simulink model "CTR_Control_Simulation"  (R2018b)
settings: Solver=FixedStepAuto  StartTime=0.0  StopTime=20  FixedStep=0.05  RelTol=1e-3
libraries: simulink x1, dspinverses x1, powerlib_meascontrol x1
settings Model: Creator=mohsen  LastModifiedBy=Mohsen
settings SFSimCC: SimUseLocalCustomCode=off
settings RTWCC: RTWUseLocalCustomCode=off

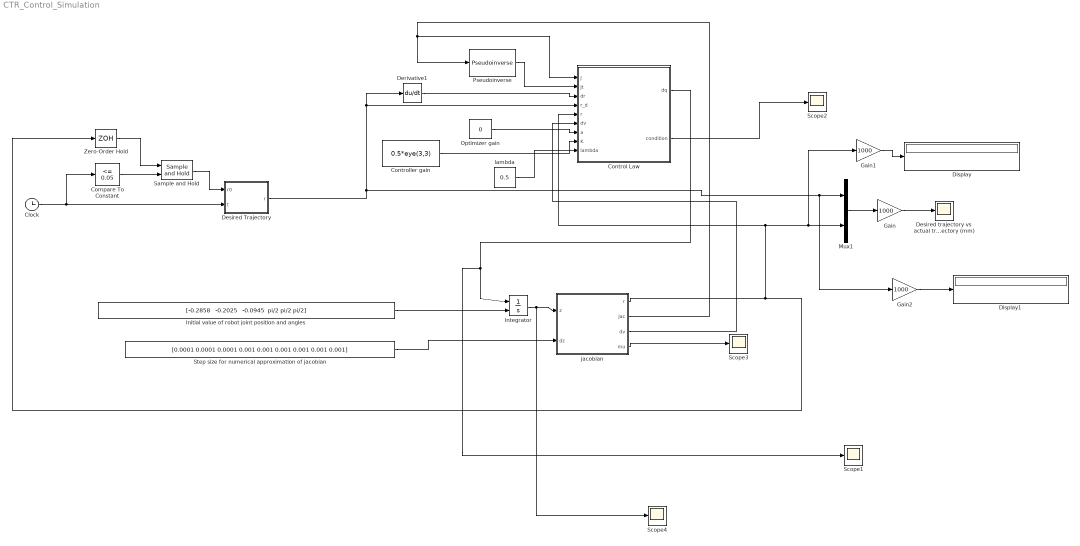
== system CTR_Control_Simulation ==
  Clock : Clock
  Compare To Constant : simulink/Logic and Bit Operations/Compare To Constant  relop=<=  const=0.05  OutDataTypeStr=boolean
  Control Law : MATLAB Function  TreatAsAtomicUnit=on
  Controller gain : Constant  Value=0.5*eye(3,3)
  Derivative1 : Derivative
  Desired Trajectory : MATLAB Function  TreatAsAtomicUnit=on
  Desired trajectory vs actual trajectory (mm) : Scope
  Display : Display
  Display1 : Display
  Gain : Gain  Gain=1000
  Gain1 : Gain  Gain=1000
  Gain2 : Gain  Gain=1000
  Initial value of robot joint position and angles : Constant  Value="[-0.2858   -0.2025   -0.0945  pi/2 pi/2 pi/2]"  VectorParams1D=off  SampleTime=-1
  Integrator : Integrator  InitialConditionSource=external  InitialCondition="[-0.2700   -0.1950   -0.0950    pi/2 pi/2 pi/2 ]"
  Mux1 : Mux  Inputs=2
  Optimizer gain : Constant  Value=0
  Pseudoinverse : dspinverses/Pseudoinverse  wanterr=off  SimulateUsing=Interpreted execution
      settings: SourceProductName=DSP System Toolbox  SourceProductBaseCode=DS
  Sample and Hold : powerlib_meascontrol/Additional Components/Sample and Hold  ic=0  Ts=0
      settings: SourceProductName=Simscape Electrical  SourceProductBaseCode=PS
  Scope{1..4} (4 alike) : Scope
  Step size for numerical approximation of jacobian : Constant  Value=[0.0001 0.0001 0.0001 0.001 0.001 0.001 0.001 0.001 0.001]
  Zero-Order Hold : ZeroOrderHold  SampleTime=5
  jacobian : MATLAB Function  TreatAsAtomicUnit=on
  lambda : Constant  Value=0.5
  wires:
  jacobian/2(Jac) -> Pseudoinverse/1, Control Law/1(J)
  Derivative1/1 -> Control Law/3(dr)
  Mux1/1 -> Gain/1
  Desired Trajectory/1(r) -> Control Law/4(r_d), Derivative1/1, Gain2/1, Mux1/1
  jacobian/1(r) -> Gain1/1, Mux1/2, Control Law/5(r), Zero-Order Hold/1
  Gain/1 -> Desired trajectory vs actual trajectory (mm)/1
  Pseudoinverse/1 -> Control Law/2(Jt)
  Control Law/1(dq) -> Scope1/1, Integrator/1
  Integrator/1 -> Scope4/1, jacobian/1(z)
  Step size for numerical approximation of jacobian/1 -> jacobian/2(dz)
  jacobian/3(dv) -> Control Law/6(dv)
  Optimizer gain/1 -> Control Law/7(a)
  jacobian/4(mu) -> Scope3/1
  Sample and Hold/1 -> Desired Trajectory/1(r0)
  Initial value of robot joint position and angles/1 -> Integrator/2
  Controller gain/1 -> Control Law/8(K)
  Clock/1 -> Compare To Constant/1, Desired Trajectory/2(t)
  Zero-Order Hold/1 -> Sample and Hold/1
  Compare To Constant/1 -> Sample and Hold/2
  Control Law/2(condition) -> Scope2/1
  lambda/1 -> Control Law/9(lambda)
  Gain1/1 -> Display/1
  Gain2/1 -> Display1/1

== matlab function CTR_Control_Simulation/Desired Trajectory ==
  data: r0 input; r output; t input
function r = fcn(r0, t)


if t>0.01
    %straight line -- set runtime to 5 sec and optimazer gain to 0.02 and
    %controller gain to 5*eye(3,3) and all inital angles to 0
    %Velocity=0.001;
    %r=r0+[-Velocity*t 2.*Velocity*t Velocity*t]';  
    
    %circle -- set runtime to 40 sec and optimazer gain to 0.02 and
    %controller gain to 2*eye(3,3) and all inital angles to pi/2
     R=0.03;            
     x=R*sin((2*pi/20)*t);
     y=R-R*cos((2*pi/20)*t);
     r=r0+[x y 0]';  
%     
%     x=0.01-0.01.*cos(t*2*pi);
%     y=0.01.*sin(t*2*pi);
%     z=0.1.*(t);
%     r=r0+[x y z]'; 
else
    
    r=r0;
end



end

== matlab function CTR_Control_Simulation/jacobian ==
  data: z input; r output; Jac output; dv output; dz input; mu output
function [r, Jac, dv, mu] = jacobian(z, dz)

% length of tubes
l=1e-3.*[328+103  219+113 174];
% length of the curved part of tubes
l_k=1e-3*[103 113 174-40];

if (iscolumn(z))
    Z=z';
else
    Z=z;
end

% initial value of twist
uz_0=[0 0 0];

% uncomment this section if you intend to include the BVP approximation of
% jacobian

% cost=ones(3,1);
% k=1;
% End=zeros(1,100); uz0_optim=zeros(3,100); a=1;
% while (sum(cost.^2))>1e-4 && k<100
%     End(k)=sum(cost.^2);
%     uz0_optim(:,k)=uz_0';
%     [cost,J] = COST(uz_0,z,l,l_k);
%     d=-J\cost;
%     a=0.4;
%     uz_0=uz_0+a*d;
%     k=k+1;
% end
% [min_error,index]=min(End(End>0));
% uz_0=uz0_optim(:,index)';
% 
% [r1,~] = moving_CTR_nmpc(Z,uz0,l,l_k);
% r=r1(end,:)';
uz0=uz_0;


[r0,~] =  moving_CTR_nmpc(z,uz0,l,l_k); 
r0=r0(end,:)';
r=r0;

Jac=zeros(3,6);
for i=1:6
    Dz=Z;
    Dz(i)=Z(i)+dz(i); 
    [dr,~] =  moving_CTR_nmpc(Dz(1:6),uz0,l,l_k); 
    Jac(:,i)=(dr(end,:)'-r0)/dz(i);
end

% penalizing jacobian columns as a function of joint limits
qmin=[-0.3 Z(1)+0.055 Z(2)+0.068];  %lower limit
qmax=[Z(2)-0.055 Z(3)-0.068 -0.015];  %upper limit

%%uncomment if you wish to penalize jacobian
% kc=1; 
% PP=[0 0 0];
% for i=1:3
% p= (1 - exp( (-4 *kc * ( Z(i)- qmin(i) ) * (qmax(i) -Z(i)) )/ (qmax(i)-qmin(i))^2 ) ) /...
%     (1-exp(-kc));
% 
%  Jac(:,i)=p.*Jac(:,i);
% PP(i)= p;
% end

% for i=4:6
% p= 1;
% 
% Jac(:,i)=p.*Jac(:,i);
% end

% estimating gradient of cost function (manipulability re-shaping)
dJac=zeros(3,6,6);
for i=1:6
    Dz=Z;
    Dz(i)=Z(i)+dz(i);
    [r0,~] =  moving_CTR_nmpc(Dz(1:6),uz0,l,l_k);  
    dr0=r0(end,:)';
for j=1:6
    DDz=Dz;
    DDz(j)=Dz(j)+dz(j); 
    [dr,~] =  moving_CTR_nmpc(DDz(1:6),uz0,l,l_k); 
    dJac(:,j,i)=(dr(end,:)'-dr0)/dz(j);
end
end
Mu_d=eye(3,3);
dv=zeros(6,1);
for i=1:6
A=(dJac(:,:,i)*dJac(:,:,i)');
Mu= A'*(A*A')^(-1);
dv(i)=log(det( (Mu+Mu_d) /2)) -0.5* log(det( Mu*Mu_d));
end

mu=sqrt(det(Jac*Jac'));
end

%% Cost function for bvp
function [cost, J] = COST(uz_0,z,l,l_k)
Wuz=1*eye(3,3);  

if ~(iscolumn(uz_0))
    uz0=uz_0';
else
    uz0=uz_0;
end

if (iscolumn(z))
    Z=z';
else
    Z=z;
end

duz0=0.001;
dz=[0 0 0 0 0 0 duz0 duz0 duz0];
[~,Uz0] =  moving_CTR_nmpc(Z,uz0',l,l_k); 
J=zeros(3,3);
Z=[Z uz_0'];

for i=7:9
    Dz=Z;
    Dz(i)=Z(i)+dz(i); 
    [~,dUz] =  moving_CTR_nmpc(Dz(1:6),Dz(7:9)',l,l_k); 
    J(:,i-6)= (dUz-Uz0)/dz(i);
end

if ~(iscolumn(Uz0))
    Uz_0=Uz0';
else
    Uz_0=Uz0;
end


cost=Wuz*Uz_0;
end


%% main ode solver
function [r1,Uz] = moving_CTR_nmpc(q,uz_0,l,l_k)

 E=[ 6.4359738368e+10,5.2548578304e+10,4.7163091968e+10];
 J= 1.0e-11 *[ 0.0120    0.0653    0.1686];
 I= 1.0e-12 *[ 0.0601    0.3267    0.8432 ];
 G=[2.5091302912e+10,2.1467424256e+10,2.9788923392e+10]; 
 Ux=[21.3 13.108 3.5];
 Uy=[0 0 0];
 n=3;
 
% q1 o q3 are robot base movments, q3 to q6 are rbot base rotation angle.

if ~(iscolumn(uz_0))
    uz0=uz_0';
else
    uz0=uz_0;
end

B=[q(1)  q(2)  q(3)];  % length of tubes before template
%initial angles

alpha=[q(4) q(5) q(6)]-B.*uz0';
alpha_1=alpha(1);

% segmenting tubes  
% check all inputs must have n elements, n is number of tubes
[L,d_tip,EE,UUx,UUy] = segmenting(E,Ux,Uy,l,B,l_k);

SS=L;
for i=1:length(L)
    SS(i)=sum(L(1:i));
%     plot((B(1)+SS(i))*ones(1,10),1:10,'b' ,'LineWidth',2)
end

% S is segmented abssica of tube after template
 S=SS(SS+min(B)>0)+min(B);
 E=zeros(n,length(S)); Ux=E; Uy=E;
 for i=1:n
    E(i,:)=EE(i,SS+min(B)>0); Ux(i,:)=UUx(i,SS+min(B)>0); Uy(i,:)=UUy(i,SS+min(B)>0);
 end
 % each (i,j) element of above matrices correspond to the jth segment of
 % ith tube, 1st tube is the most inner

 %% Solving ode for shape

span=[0 S];       % vector of tube abssica starting at zero
Length=[]; r=[]; U_z=[]; % solved length, curvatures, and twist angles
%U1_after=[0;0;0];             % 1st tube initial curvature at segment beginning
r0=[ 0 0 0]'; R0=[cos(alpha_1) sin(alpha_1) 0; -sin(alpha_1) cos(alpha_1) 0; 0 0 1];
R0=reshape(R0,[9,1]);
%alpha=alpha-B.*uz_0'; 

for seg=1:length(S)
    
s_span = [span(seg) span(seg+1)-0.0000001];
y0_1=[r0 ; R0];

y0_2=zeros(2*n,1);
y0_2(n+1:2*n)=alpha;
y0_2(1:n)=uz0;

y_0=[y0_2; y0_1];

[s,y] = ode23(@(s,y) ode5(s,y,Ux(:,seg),Uy(:,seg),E(:,seg).*I',G.*J,n), s_span, y_0);
% first n elements of y are curvatures along z, e.g., y= [ u1_z  u2_z ... ]
% last n elements of y are twist angles, alpha_i
shape=[y(:,2*n+1),y(:,2*n+2),y(:,2*n+3)];
Length=[Length; s];
r=[r; shape];
U_z=[U_z; y(:,1:n )];
r0=shape(end,:)';
R0=y(end,2*n+4:2*n+12)';
uz0=U_z(end,:)';

end

Uz=zeros(n,1);
for i=1:n
[~,index] =  min( abs(Length-d_tip(i)+0.0001) );
Uz(i)= U_z(index,i);
end

r1=r;

end


%% ODE
function dydt = ode5(~,y,Ux,Uy,EI,GJ,n)

dydt=zeros(2*n+12,1);
% first n elements of y are curvatures along z, e.g., y= [ u1_z  u2_z ... ]
% second n elements of y are twist angles, alpha_i
% last 12 elements are r (position) and R (orientations), respectively


% calculating 1st tube's curvatures in x and y direction
ux=zeros(n,1);uy=zeros(n,1);

% calculating tube's curvatures in x and y direction
for i=1:n  
ux(i)= (1/(EI(1)+EI(2)+EI(3)))* (...
      EI(1)*Ux(1)*cos(y(n+i)-y(n+1))+ EI(1)*Uy(1)*sin(y(n+i)-y(n+1))  + ...
      EI(2)*Ux(2)*cos(y(n+i)-y(n+2))+ EI(2)*Uy(2)*sin(y(n+i)-y(n+2))  + ...
      EI(3)*Ux(3)*cos(y(n+i)-y(n+3))+ EI(3)*Uy(3)*sin(y(n+i)-y(n+3)) );
uy(i)= (1/(EI(1)+EI(2)+EI(3)))* (...
      -EI(1)*Ux(1)*sin(y(n+i)-y(n+1))+ EI(1)*Uy(1)*cos(y(n+i)-y(n+1))  + ...
      -EI(2)*Ux(2)*sin(y(n+i)-y(n+2))+ EI(2)*Uy(2)*cos(y(n+i)-y(n+2))  + ...
      -EI(3)*Ux(3)*sin(y(n+i)-y(n+3))+ EI(3)*Uy(3)*cos(y(n+i)-y(n+3)) ); 
end

% odes for twist
for i=1:n      
    dydt(i)=  (  (EI(i))/(GJ(i))  ) * ( ux(i)* Uy(i) -  uy(i)* Ux(i) );  % ui_z
    dydt(n+i)=  y(i);   %alpha_i
end


e3=[0 0 1]';              
uz = y(1:n); 



% y(1) to y(3) are position of point materials
%r1=[y(1); y(2); y(3)];
% y(4) to y(12) are rotation matrix elements
R1=[y(2*n+4) y(2*n+5) y(2*n+6);y(2*n+7) y(2*n+8) y(2*n+9);y(2*n+10) y(2*n+11) y(2*n+12)];


u_hat=[0 -uz(1) uy(1) ; uz(1) 0 -ux(1) ; -uy(1) ux(1) 0 ];


% odes
dr1 = R1*e3;
dR1=R1*u_hat;


dydt(2*n+1)=dr1(1);dydt(2*n+2)=dr1(2);dydt(2*n+3)=dr1(3);
dR=dR1'; 
dR=dR(:);
for i=4:12
   dydt(2*n+i)=dR(i-3);
end

end


%% code for segmenting tubes
function [L,d1,E,Ux,Uy,I,G,J] = segmenting(E,Ux,Uy,l,B,l_k)

% all vectors must be sorted, starting element belongs to the most inner tube
%E, U, I, G, J   stifness, curvature, inertia, torsion constant, and second moment of inertia vectors for each tube
%l vector of tube length
%B  vector of tube movments with respect to template position, i.e., s=0 (always negative)
%l_k vecot oftube's curved part length


d1= l+B; % position of tip of the tubes
d2=d1-l_k; % position of the point where tube bending starts
points=[0 B d2 d1];
[L, index]=sort(points);
L = 1e-5*floor(1e5*diff(L));  % length of each segment 
%(used floor because diff command doesn't give absolute zero sometimes)
% 
% for i=1:k-1
% if B(i)>B(i+1)
%     sprintf('inner tube is clashing into outer tubes')
%     E=zeros(k,length(L));
%     I=E; G=E; J=E; Ux=E; Uy=E;
%     return
% end
% end

EE=zeros(3,length(L));
II=EE; GG=EE; JJ=EE; UUx=EE; UUy=EE;

for i=1:3

[~, a] = min(abs(index-i+1)); % find where tube begins
[~, b] = min(abs(index-(1*3+i+1))); % find where tube curve starts
[~, c] = min(abs(index-(2*3+i+1))); % find where tube ends

if L(a)==0; a=a+1;  end
if L(b)==0; b=b+1;  end
if c<=length(L)
    if L(c)==0; c=c+1; end
end
    
EE(i,a:c-1)=E(i);
UUx(i,b:c-1)=Ux(i);
UUy(i,b:c-1)=Uy(i);
end

l=L(~(L==0));  % get rid of zero lengthes
E=zeros(3,length(l)); Ux=E; Uy=E;
 for i=1:3
    E(i,:)=EE(i,~(L==0)); Ux(i,:)=UUx(i,~(L==0)); Uy(i,:)=UUy(i,~(L==0));
 end
L=L(~(L==0));

end

== matlab function CTR_Control_Simulation/Control Law ==
  data: J input; Jt input; dq output; dr input; r_d input; r input; dv input; a input; K input; condition output; lambda input
function [dq , condition] = fcn(J, Jt,dr, r_d,r, dv, a, K,lambda)

coder.extrinsic('cond');

condition=0;

dq = Jt*(dr + K*(r_d-r) ) - a* (eye(6,6)- Jt*J)*dv;


% for damped-least squared jacobian
J_d=inv(Jt*J+lambda^2*eye(6,6))*Jt;
dq = J_d*(dr + K*(r_d-r) ) ;

condition=cond(Jt);
